simulink model "SimpleTransmission_R2022a"  (R2022a)
settings: Solver=VariableStepAuto  StartTime=0.0  StopTime=100  RelTol=1e-3
values from neighbouring files (symbols this model uses):
  len = length(seq)    [help_cod.m]
  len2 = length(array)    [help_cod.m]
  seq = sequence.'    [help_cod.m]
libraries: dspsrcs4 x4, simulink x3, commsequence2 x3, dspsigops x3, commdigbbndpm3 x2, commfilt2 x2, commchan3 x1, commrflib2 x1, commsink2 x1, commsync2 x1
settings Model: PacingRate=0.001000  Creator=svdvl  LastModifiedBy=Владислав
settings ModelReferenceCC: EnableRefExpFcnMdlSchedulingChecks=off
settings RTWCC: Description=Generic Real-Time Target

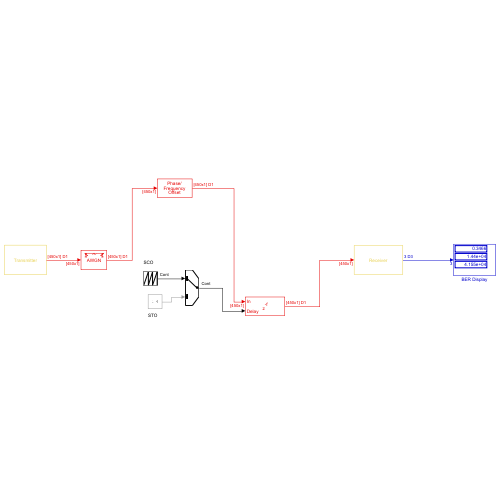
[thumbnail: Simulink's stored preview of the top-level diagram]
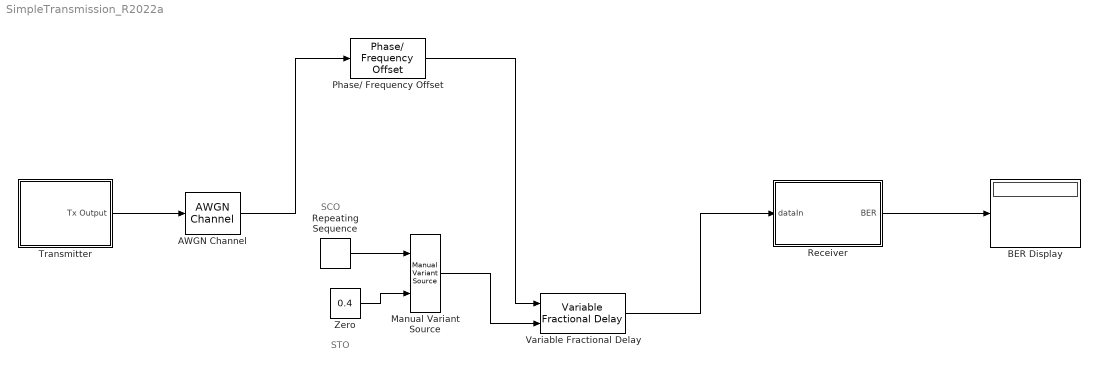
== system SimpleTransmission_R2022a ==
  note: STO
  note: SCO
  AWGN Channel : commchan3/AWGN Channel  InputProcessing=Columns as channels (frame based)  seed=1  noiseMode="Signal to noise ratio  (SNR)"  EbNodB=4  EsNodB=20  SNRdB=20  bitsPerSym=2  Ps=0.5  Tsym=2e-5  variance=1
  BER Display : Display
  Manual Variant Source : simulink/Signal Routing/Manual Variant Source  NumChoices=2  LabelModeActiveChoice=V_1
  Phase/ Frequency Offset : commrflib2/Phase// Frequency Offset  phaseOffset=0  freqPort=off  freqOffset=-50
  Receiver : Subsystem
      mask Display: disp('Receiver')
  Repeating Sequence : simulink/Sources/Repeating Sequence  rep_seq_t=[0 0.0001]  rep_seq_y=[0 0.9]
  Transmitter : Subsystem
      mask Display: disp('Transmitter')
  Variable Fractional Delay : dspsigops/Variable Fractional Delay  mode=OBSOLETE  modeActive=Linear  L=4  FarrowL=4  R=10  alpha=1  dmax=65000  InputProcessing=Columns as channels (frame based)  ic=0  noDFT=off  fallbackFIR=Clip to the minimum value necessary for centered kernel  fallbackFarrow=Clip to the minimum value necessary for centered kernel  roundingMode=Zero  overflowMode=off
      settings: SourceProductBaseCode=DS
  Zero : Constant  Value=0.4  VectorParams1D=off  OutDataTypeStr=double  SampleTime=-1
  wires:
  Transmitter/1(Tx Output) -> AWGN Channel/1
  Receiver/1(BER) -> BER Display/1
  Repeating Sequence/1 -> Manual Variant Source/1
  Zero/1 -> Manual Variant Source/2
  Manual Variant Source/1 -> Variable Fractional Delay/2
  Phase/ Frequency Offset/1 -> Variable Fractional Delay/1
  AWGN Channel/1 -> Phase/ Frequency Offset/1
  Variable Fractional Delay/1 -> Receiver/1(dataIn)

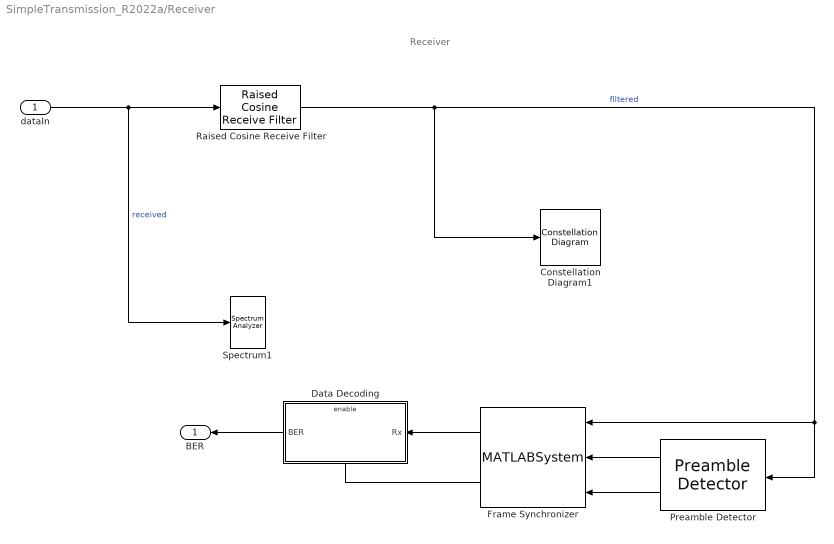
== system SimpleTransmission_R2022a/Receiver ==
  note: Receiver
  dataIn : Inport
  Constellation Diagram1 : ConstellationDiagram  WindowPosition=[67.000000,341.000000,601.000000,434.000000,]  Visible=on  ScopeFrameLocation=window  SymbolsToDisplaySource=Property  SymbolsToDisplay=500  XLimits=[-2.18,2.18]  YLimits=[-1.38,1.38]
  Data Decoding : Subsystem
      mask Display: disp('Data Decoding');
  Frame Synchronizer : MATLABSystem  System=FrameSynchronizer  Input=Symbol  OutputFrameLength=fix((len*2+len2)/2)  PreambleLength=len  SimulateUsing=Code generation
      mask Type: FrameSynchronizer
      mask Display:
      | disp(['Frame' char(10) 'Synchronizer']);
      | port_label('input',1,'u');
      | port_label('input',2,'idx');
      | port_label('input',3,'dtMt');
      | port_label('output',1,'Frame');
      | port_label('output',2,'Valid');
  Preamble Detector : commsync2/Preamble Detector  Input=Symbol  Preamble=sqrt(2)/2 * (-1-1i) * (seq)  Threshold=8  DetectionMetricOutput=on  Detections=All  SimulateUsing=Code generation
      settings: SourceProductBaseCode=CM
  Raised Cosine Receive Filter : commfilt2/Raised Cosine Receive Filter  filtType=Square root  R=0.5  filtSpan=12  N=2  downFactor=2  downOffset=0  filterGain=1  InputProcessing=Columns as channels (frame based)  RateOptions=Enforce single-rate processing  framing=Mute  checkCoeff=off  variableName=rcRxFilt  currentFiltSpan=10  D=5  inputOffset=0  sampMode=Mute  saveAsFlag=0  rateMode=Downsampling  checkGain=Normalized  launchFVT=on  roundingMode=Floor  overflowMode=off  coeffDataTypeStr=Inherit: Same word length as input  coeffMin=[]  coeffMax=[]  coeffLastDataTypeStr=Inherit: Same word length as input  accumDataTypeStr=Inherit: Same as product output  accumLastDataTypeStr=Inherit: Same as product output  outputDataTypeStr=Inherit: Same as accumulator  outputMin=[]  outputMax=[]  outputLastDataTypeStr=Inherit: Same as accumulator
  Spectrum1 : SpectrumAnalyzer
  BER : Outport  VectorParamsAs1DForOutWhenUnconnected=off
  wires:
  Raised Cosine Receive Filter/1 -> Constellation Diagram1/1, Preamble Detector/1, Frame Synchronizer/1  "filtered"
  dataIn/1 -> Spectrum1/1, Raised Cosine Receive Filter/1  "received"
  Frame Synchronizer/1 -> Data Decoding/1(Rx)
  Preamble Detector/1 -> Frame Synchronizer/2
  Frame Synchronizer/2 -> Data Decoding/Enable
  Data Decoding/1(BER) -> BER/1
  Preamble Detector/2 -> Frame Synchronizer/3

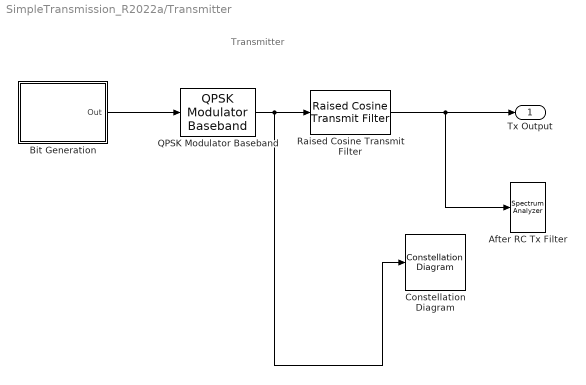
== system SimpleTransmission_R2022a/Transmitter ==
  note: Transmitter
  After RC Tx Filter : SpectrumAnalyzer
  Bit Generation : Subsystem
      mask Display: disp('Bits Generation')
  Constellation Diagram : ConstellationDiagram  WindowPosition=[40.000000,31.000000,504.000000,324.000000,]  Visible=on  ScopeFrameLocation=window
  QPSK Modulator Baseband : commdigbbndpm3/QPSK Modulator Baseband  InType=Bit  Enc=Gray  Ph=pi/4  outDtype=double  outWordLen=16  outUDDataType=sfix(16)  outFracLenMode=Best precision  outFracLen=15  outDataTypeStr=double  outLastDataTypeStr=double
  Raised Cosine Transmit Filter : commfilt2/Raised Cosine Transmit Filter  filtType=Square root  R=0.5  filtSpan=12  N=2  filterGain=1  InputProcessing=Columns as channels (frame based)  RateOptions=Enforce single-rate processing  framing=Mute  checkCoeff=off  variableName=rcTxFilt1  checkGain=Normalized  sampMode=Mute  saveAsFlag=0  currentFiltSpan=10  D=5  launchFVT=on  roundingMode=Floor  overflowMode=off  coeffDataTypeStr=Inherit: Same word length as input  coeffMin=[]  coeffMax=[]  coeffLastDataTypeStr=Inherit: Same word length as input  outputDataTypeStr=Inherit: Same as accumulator  outputMin=[]  outputMax=[]  outputLastDataTypeStr=Inherit: Same as accumulator
  Tx Output : Outport  VectorParamsAs1DForOutWhenUnconnected=off
  wires:
  Raised Cosine Transmit Filter/1 -> Tx Output/1, After RC Tx Filter/1
  Bit Generation/1(Out) -> QPSK Modulator Baseband/1
  QPSK Modulator Baseband/1 -> Constellation Diagram/1, Raised Cosine Transmit Filter/1

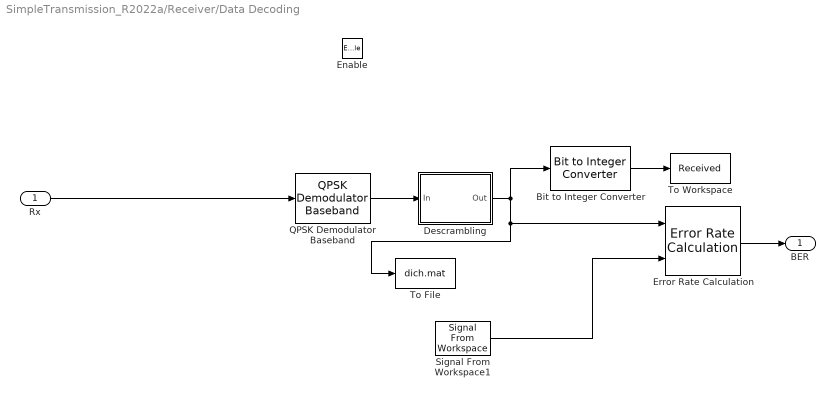
== system SimpleTransmission_R2022a/Receiver/Data Decoding ==
  Rx : Inport
  Enable : EnablePort
  Bit to Integer Converter : simulink/Logic and Bit Operations/Bit to Integer Converter  nbits=maxdev  bitOrder=MSB first  signedOutputValues=Unsigned  outDtype=Inherit via internal rule  outDtypeSigned=Inherit via internal rule
      settings: SourceProductBaseCode=SL
  Descrambling : Subsystem
      mask Display: disp('Descrambling');
  Error Rate Calculation : commsink2/Error Rate Calculation  N=0  st_delay=0  cp_mode=Entire frame  subframe=ans.BerMask  PMode=Port  WsName=ErrorVec  RsMode2=off  stop=off  numErr=100  maxBits=1e6
  QPSK Demodulator Baseband : commdigbbndpm3/QPSK Demodulator Baseband  OutType=Bit  DecType=Hard decision  VarSource=Dialog  Variance=1  Dec=Gray  Ph=pi/4  outDtype1=Inherit via internal rule  outDtype2=Inherit via internal rule  derotateFactorWordLen=16  derotateFactorDataTypeStr=Inherit: Same word length as input  derotateFactorLastDataTypeStr=Inherit: Same word length as input
  Signal From Workspace1 : dspsrcs4/Signal From Workspace  X=array.'  Ts=1.0116e-05  nsamps=len2  OutputAfterFinalValue=Cyclic repetition  ignoreOrWarnInputAndFrameLengths=on  OutputFrames=off
  To File : ToFile  Filename=dich.mat
  To Workspace : ToWorkspace  VariableName=Received  SaveFormat=Structure  SampleTime=-1
      settings: Save2DSignal=2-D array (concatenate along first dimension)
  BER : Outport  VectorParamsAs1DForOutWhenUnconnected=off
  wires:
  Rx/1 -> QPSK Demodulator Baseband/1
  Error Rate Calculation/1 -> BER/1
  QPSK Demodulator Baseband/1 -> Descrambling/1(In)
  Bit to Integer Converter/1 -> To Workspace/1
  Signal From Workspace1/1 -> Error Rate Calculation/2
  Descrambling/1(Out) -> Bit to Integer Converter/1, To File/1, Error Rate Calculation/1

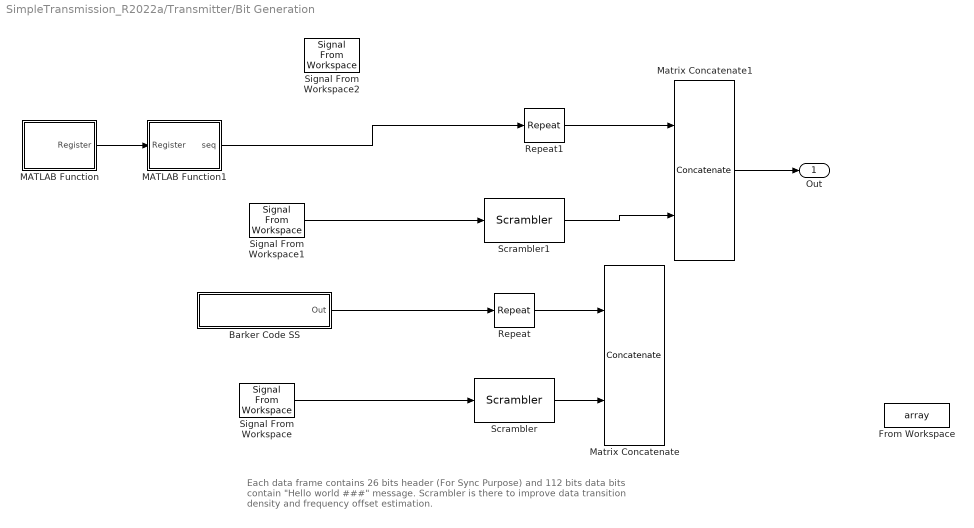
== system SimpleTransmission_R2022a/Transmitter/Bit Generation ==
  note: Each data frame contains 26 bits header (For Sync Purpose) and 112 bits data bits
      | contain "Hello world ###" message. Scrambler is there to improve data
      | transition density and frequency offset estimation.
  Barker Code SS : Subsystem
      mask Display: disp('Unipolar\nBarker Code')
  From Workspace : FromWorkspace  VariableName=array
  MATLAB Function : MATLAB Function  TreatAsAtomicUnit=on
  MATLAB Function1 : MATLAB Function  TreatAsAtomicUnit=on
  Matrix Concatenate : Concatenate  Mode=Multidimensional array
  Matrix Concatenate1 : Concatenate  Mode=Multidimensional array
  Repeat : dspsigops/Repeat  N=2  InputProcessing=Columns as channels (frame based)  RateOptions=Enforce single-rate processing  ic=0  mode=Unused parameter value
  Repeat1 : dspsigops/Repeat  N=2  InputProcessing=Columns as channels (frame based)  RateOptions=Enforce single-rate processing  ic=0  mode=Unused parameter value
  Scrambler : commsequence2/Scrambler  M=2  poly=[1 1 1 0 1]  iniStaSource=Dialog Parameter  ini_sta=[1 0 0 0]  resetViaPort=off
      settings: SourceProductBaseCode=CM
  Scrambler1 : commsequence2/Scrambler  M=2  poly=[1 1 1 0 1]  iniStaSource=Dialog Parameter  ini_sta=[1 0 0 0]  resetViaPort=off
      settings: SourceProductBaseCode=CM
  Signal From Workspace : dspsrcs4/Signal From Workspace  X="[1\t0\t0\t1\t0\t0\t0\t1\t1\t0\t0\t1\t0\t1\t1\t1\t0\t1\t1\t0\t0\t1\t1\t0\t1\t1\t0\t0\t1\t1\t0\t1\t1\t1\t1\t0\t1\t0\t0\t0\t0\t0\t1\t1\t1\t0\t1\t1\t1\t1\t1\t0\t1\t1\t1\t1\t1\t1\t1\t0\t0\t1\t0\t1\t1\t0\t1\t1\t0\t0\t1\t1\t0\t0\t1\t0\t0\t0\t1\t0\t0\t0\t0\t0\t0\t1\t1\t0\t0\t0\t0\t0\t1\t1\t0\t0\t0\t0\t0\t1\t1\t0\t0\t0\t0\t0\t0\t0\t1\t0\t1\t0\t1\t0\t0\t1\t0\t0\t0\t1\t1\t0\t0\t1\t0\t1\t1\t1\t0\t1\t1\t0\t0\t1 ...(+33198 chars)].'"  Ts=1.0116e-05  nsamps=2240  OutputAfterFinalValue=Cyclic repetition  ignoreOrWarnInputAndFrameLengths=on  OutputFrames=off
  Signal From Workspace1 : dspsrcs4/Signal From Workspace  X=array.'  Ts=1.0116e-05  nsamps=len2  OutputAfterFinalValue=Cyclic repetition  ignoreOrWarnInputAndFrameLengths=on  OutputFrames=off
  Signal From Workspace2 : dspsrcs4/Signal From Workspace  X=scrseq  Ts=1.0116e-05  nsamps=len  OutputAfterFinalValue=Cyclic repetition  ignoreOrWarnInputAndFrameLengths=on  OutputFrames=off
  Out : Outport  VectorParamsAs1DForOutWhenUnconnected=off
  wires:
  Barker Code SS/1(Out) -> Repeat/1
  Repeat/1 -> Matrix Concatenate/1
  Scrambler/1 -> Matrix Concatenate/2
  Signal From Workspace/1 -> Scrambler/1
  MATLAB Function/1(Register) -> MATLAB Function1/1(Register)
  Repeat1/1 -> Matrix Concatenate1/1
  Signal From Workspace1/1 -> Scrambler1/1
  Scrambler1/1 -> Matrix Concatenate1/2
  Matrix Concatenate1/1 -> Out/1
  MATLAB Function1/1(seq) -> Repeat1/1

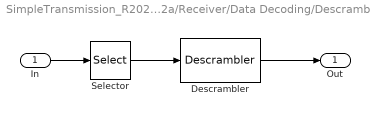
== system SimpleTransmission_R2022a/Receiver/Data Decoding/Descrambling ==
  In : Inport
  Descrambler : commsequence2/Descrambler  M=2  poly=[1 1 1 0 1]  iniStaSource=Dialog Parameter  ini_sta=[1 0 0 0]  resetViaPort=off
      settings: SourceProductBaseCode=CM
  Selector : Selector  IndexOptions=Index vector (dialog)  Indices=[(2*len+1):(len*2+len2)]  OutputSizes=1
  Out : Outport  VectorParamsAs1DForOutWhenUnconnected=off
  wires:
  In/1 -> Selector/1
  Selector/1 -> Descrambler/1
  Descrambler/1 -> Out/1

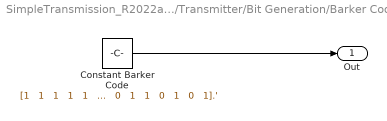
== system SimpleTransmission_R2022a/Transmitter/Bit Generation/Barker Code SS ==
  Constant Barker Code : Constant  Value="[1   1   1   1   1   0   0   1   1   0   1   0   1].'"  VectorParams1D=off  OutDataTypeStr=double
  Out : Outport  VectorParamsAs1DForOutWhenUnconnected=off
  wires:
  Constant Barker Code/1 -> Out/1

== matlab function SimpleTransmission_R2022a/Transmitter/Bit Generation/MATLAB Function ==
  data: Register output
function Register = fcn()
Register = [1 0 0 1 0 1 0 1 0]; % начальное состояние регистра

== matlab function SimpleTransmission_R2022a/Transmitter/Bit Generation/MATLAB Function1 ==
  data: Register input; seq output
function seq = Scrambler(Register)
    % Инициализация параметров
    %m = 8; % число бит регистра
    sequence_length = 2^7-1; % длина псевдослучайной последовательности
    sequence = zeros(1, sequence_length); % инициализация последовательности
    
    % Генерация псевдослучайной последовательности
    for i = 1:sequence_length
        sequence(i)=xor(Register(end), Register(end-1)); % выходной бит
        feedback = sequence(i); 

        Register = circshift(Register,1); % сдвиг регистра
        Register(1) = feedback; % обновление первого бита
    end
    seq=sequence.';
end
